simulink model "Q1"  (R2022b)
settings: Solver=VariableStepAuto  StartTime=0.0  StopTime=30  RelTol=1e-3
libraries: mpclib x5, slpidlib x3
settings Model: Creator=Alireza  LastModifiedBy=Alireza

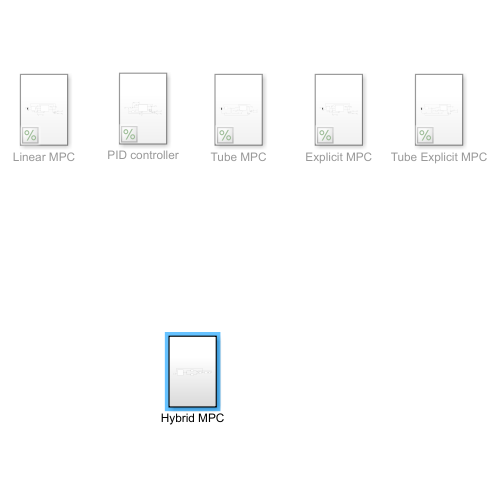
[thumbnail: Simulink's stored preview of the top-level diagram]
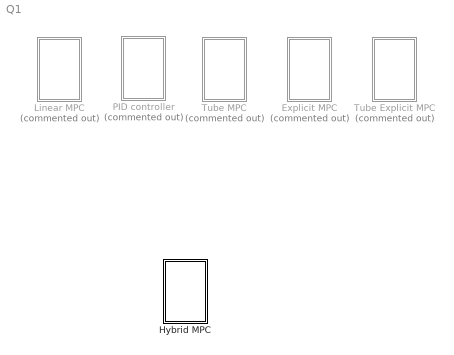
== system Q1 ==
  Explicit MPC : Subsystem  Commented=on
  Hybrid MPC : Subsystem
  Linear MPC : Subsystem  Commented=on
  PID controller : Subsystem  Commented=on
  Tube Explicit MPC : Subsystem  Commented=on
  Tube MPC : Subsystem  Commented=on

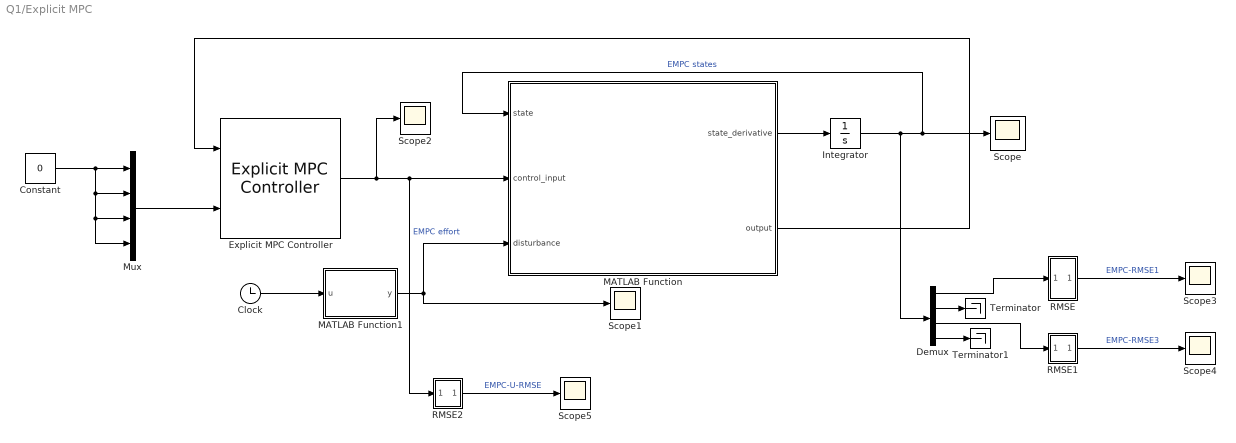
== system Q1/Explicit MPC ==
  Clock : Clock
  Constant : Constant  Value=0
  Demux : Demux
  Explicit MPC Controller : mpclib/Explicit MPC Controller  SCDEnableBlockLinearizationSpecification=on  empcobj=empc1  is_multiple=0  enable_value=0  return_u0=off  md_inport=off  mv_inport=off  return_status=off  return_region=off  return_state=off  state_inport=off  BlockDataType=double  SampleTimeInherited=off  switch_inport=off
  Integrator : Integrator  InitialCondition=[0;0;0;0]
  MATLAB Function : MATLAB Function  TreatAsAtomicUnit=on
  MATLAB Function1 : MATLAB Function  TreatAsAtomicUnit=on
  Mux : Mux
  RMSE : Subsystem
  RMSE1 : Subsystem
  RMSE2 : Subsystem
  Scope{,1..5} (6 alike) : Scope
  Terminator : Terminator
  Terminator1 : Terminator
  wires:
  RMSE/1(Out1) -> Scope3/1  "EMPC-RMSE1"
  MATLAB Function1/1(y) -> Scope1/1, MATLAB Function/3(disturbance)
  Constant/1 -> Mux/3, Mux/4, Mux/2, Mux/1
  Integrator/1 -> Demux/1, MATLAB Function/1(state), Scope/1  "EMPC states"
  Explicit MPC Controller/1 -> RMSE2/1(In1), MATLAB Function/2(control_input), Scope2/1  "EMPC effort"
  Demux/3 -> RMSE1/1(In1)
  Demux/2 -> Terminator/1
  Demux/4 -> Terminator1/1
  MATLAB Function/2(output) -> Explicit MPC Controller/1
  Demux/1 -> RMSE/1(In1)
  Mux/1 -> Explicit MPC Controller/2
  Clock/1 -> MATLAB Function1/1(u)
  MATLAB Function/1(state_derivative) -> Integrator/1
  RMSE1/1(Out1) -> Scope4/1  "EMPC-RMSE3"
  RMSE2/1(Out1) -> Scope5/1  "EMPC-U-RMSE"

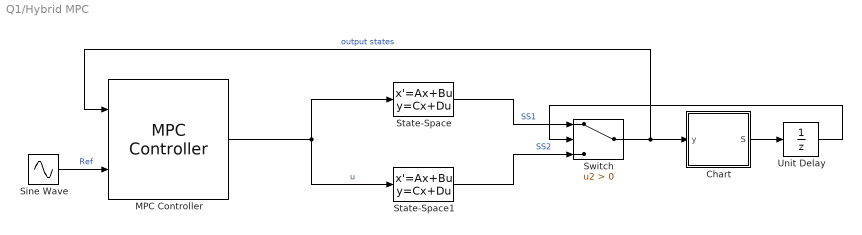
== system Q1/Hybrid MPC ==
  Chart : Stateflow chart  TreatAsAtomicUnit=on
  MPC Controller : mpclib/MPC Controller  SCDEnableBlockLinearizationSpecification=on  mpcobj=mpc1  is_multiple=0  enable_value=0  return_u0=off  updateMPCinCallerWorkspace=on  md_inport=off  mv_inport=off  uref_inport=off  return_cost=off  return_mvseq=off  return_qpstatus=off  return_xseq=off  return_state=off  return_ovseq=off  state_inport=off  umin_inport=off  umax_inport=off  ymin_inport=off  ymax_inport=off  cc_inport=off  ywt_inport=off  uwt_inport=off  duwt_inport=off  rhoeps_inport=off  pm_inport=off  MaximumP=10  HorizonChoice=FixedHorizon  n_ts=0.01  n_p=110  n_mv=1  n_md=0  n_ud=0  n_mo=1  n_uo=0  BlockDataType=double  SampleTimeInherited=off  switch_inport=off
  Sine Wave : Sin  Amplitude=20  Frequency=pi/10  SampleTime=0
  State-Space : StateSpace  A=[0 2;-2 -2]  B=[0;2]  C=[1 0]  D=[0]  InitialCondition=[0.5 ; 0]
  State-Space1 : StateSpace  A=[0 4;-4 -4]  B=[0;4]  C=[1 0]  D=[0]  InitialCondition=[0.5 ; 0]
  Switch : Switch  Criteria=u2 > Threshold  SaturateOnIntegerOverflow=off  InputSameDT=off
  Unit Delay : UnitDelay  SampleTime=-1  HasFrameUpgradeWarning=on
  wires:
  MPC Controller/1 -> State-Space1/1, State-Space/1  "u"
  State-Space1/1 -> Switch/3  "SS2"
  Switch/1 -> MPC Controller/1, Chart/1(y)  "output states"
  Sine Wave/1 -> MPC Controller/2  "Ref"
  State-Space/1 -> Switch/1  "SS1"
  Chart/1(S) -> Unit Delay/1
  Unit Delay/1 -> Switch/2

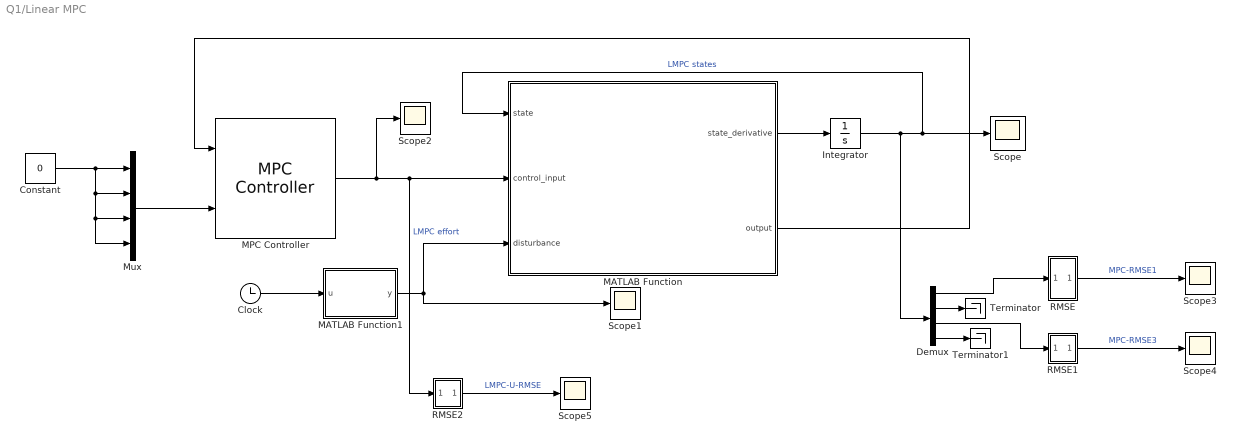
== system Q1/Linear MPC ==
  Clock : Clock
  Constant : Constant  Value=0
  Demux : Demux
  Integrator : Integrator  InitialCondition=[0;0;0;0]
  MATLAB Function : MATLAB Function  TreatAsAtomicUnit=on
  MATLAB Function1 : MATLAB Function  TreatAsAtomicUnit=on
  MPC Controller : mpclib/MPC Controller  SCDEnableBlockLinearizationSpecification=on  mpcobj=mpc1  is_multiple=0  enable_value=0  return_u0=off  updateMPCinCallerWorkspace=on  md_inport=off  mv_inport=off  uref_inport=off  return_cost=off  return_mvseq=off  return_qpstatus=off  return_xseq=off  return_state=off  return_ovseq=off  state_inport=off  umin_inport=off  umax_inport=off  ymin_inport=off  ymax_inport=off  cc_inport=off  ywt_inport=off  uwt_inport=off  duwt_inport=off  rhoeps_inport=off  pm_inport=off  MaximumP=10  HorizonChoice=FixedHorizon  n_ts=0.01  n_p=100  n_mv=1  n_md=0  n_ud=0  n_mo=4  n_uo=0  BlockDataType=double  SampleTimeInherited=off  switch_inport=off
  Mux : Mux
  RMSE : Subsystem
  RMSE1 : Subsystem
  RMSE2 : Subsystem
  Scope{,1..5} (6 alike) : Scope
  Terminator : Terminator
  Terminator1 : Terminator
  wires:
  RMSE/1(Out1) -> Scope3/1  "MPC-RMSE1"
  MATLAB Function1/1(y) -> Scope1/1, MATLAB Function/3(disturbance)
  Constant/1 -> Mux/3, Mux/4, Mux/2, Mux/1
  Integrator/1 -> Demux/1, MATLAB Function/1(state), Scope/1  "LMPC states"
  MPC Controller/1 -> RMSE2/1(In1), MATLAB Function/2(control_input), Scope2/1  "LMPC effort"
  Demux/3 -> RMSE1/1(In1)
  Demux/2 -> Terminator/1
  Demux/4 -> Terminator1/1
  MATLAB Function/2(output) -> MPC Controller/1
  Demux/1 -> RMSE/1(In1)
  Mux/1 -> MPC Controller/2
  Clock/1 -> MATLAB Function1/1(u)
  MATLAB Function/1(state_derivative) -> Integrator/1
  RMSE1/1(Out1) -> Scope4/1  "MPC-RMSE3"
  RMSE2/1(Out1) -> Scope5/1  "LMPC-U-RMSE"

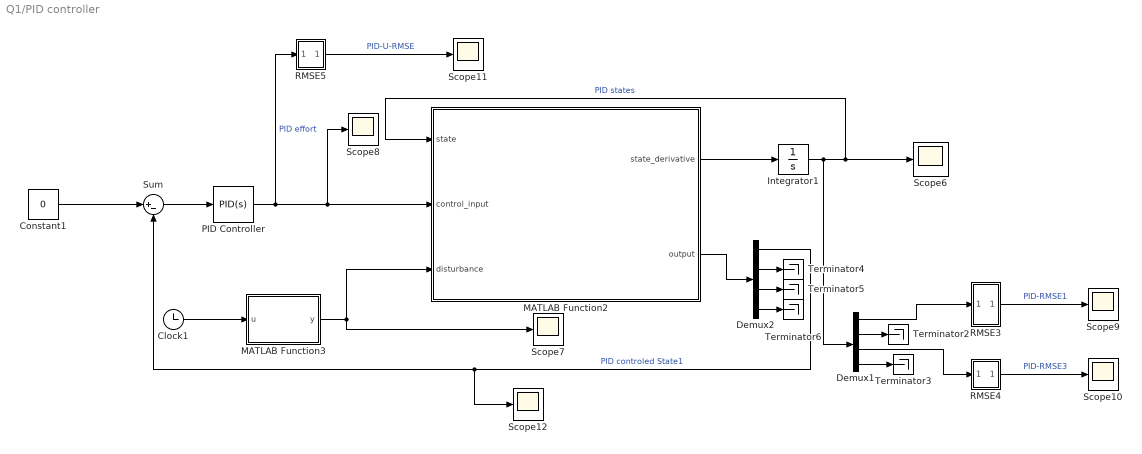
== system Q1/PID controller ==
  Clock1 : Clock
  Constant1 : Constant  Value=0
  Demux1 : Demux
  Demux2 : Demux
  Integrator1 : Integrator  InitialCondition=[0;0;0;0]
  MATLAB Function2 : MATLAB Function  TreatAsAtomicUnit=on
  MATLAB Function3 : MATLAB Function  TreatAsAtomicUnit=on
  PID Controller : slpidlib/PID Controller  Controller=PID  Form=Parallel  TimeDomain=Continuous-time  UseExternalTs=off  SampleTime=-1  IntegratorMethod=Forward Euler  FilterMethod=Forward Euler  ControllerParametersSource=internal  P=2115167.33224621  I=6808255.34812067  UseKiTs=off  D=134270.145058429  N=315.344677005256  UseFilter=on  TunerSelectOption=Transfer Function Based (PID Tuner App)  InitialConditionSource=internal  InitialConditionForIntegrator=0  InitialConditionForFilter=0  DifferentiatorICPrevScaledInput=0  ExternalReset=none  TrackingMode=off  Kt=1  LimitOutput=off  SatLimitsSource=internal  UpperSaturationLimit=inf  LowerSaturationLimit=-inf  LinearizeAsGain=on  AntiWindupMode=none  Kb=1  LimitIntegrator=off  UpperIntegratorSaturationLimit=inf  LowerIntegratorSaturationLimit=-inf  POutMin=[]  POutMax=[]  IOutMin=[]  IOutMax=[]  DOutMin=[]  DOutMax=[]  NOutMin=[]  NOutMax=[]  SumOutMin=[]  SumOutMax=[]  SaturationOutMin=[]  SaturationOutMax=[]  PParamMin=[]  PParamMax=[]  IParamMin=[]  IParamMax=[]  DParamMin=[]  DParamMax=[]  NParamMin=[]  NParamMax=[]  KbParamMin=[]  KbParamMax=[]  KtParamMin=[]  KtParamMax=[]  KbOutMin=[]  KbOutMax=[]  KtOutMin=[]  KtOutMax=[]  IntegratorOutMin=[]  IntegratorOutMax=[]  FilterOutMin=[]  FilterOutMax=[]  SumI1OutMin=[]  SumI1OutMax=[]  SumI2OutMin=[]  SumI2OutMax=[]  SumI3OutMin=[]  SumI3OutMax=[]  SumI4OutMin=[]  SumI4OutMax=[]  SumDOutMin=[]  SumDOutMax=[]  DifferentiatorOutMin=[]  DifferentiatorOutMax=[]  FilterDiffOutCoefMin=[]  FilterDiffOutCoefMax=[]  ReciprocalOutMin=[]  ReciprocalOutMax=[]  SumDenOutMin=[]  SumDenOutMax=[]  SumNumOutMin=[]  SumNumOutMax=[]  DivideOutMin=[]  DivideOutMax=[]  UdiffTsProdOutMin=[]  UdiffTsProdOutMax=[]  NTsProdOutMin=[]  NTsProdOutMax=[]  UintegralTsProdOutMin=[]  UintegralTsProdOutMax=[]  UngainTsProdOutMin=[]  UngainTsProdOutMax=[]  ClampingZeroOutDataTypeStr=Inherit: Inherit via back propagation  ClampingZeroOutMin=[]  ClampingZeroOutMax=[]  FilterDenConstantOutDataTypeStr=Inherit: Inherit via back propagation  FilterDenConstantOutMin=[]  FilterDenConstantOutMax=[]  PCopyOutDataTypeStr=Inherit: Inherit via back propagation  PCopyOutMin=[]  PCopyOutMax=[]  NCopyOutDataTypeStr=Inherit: Inherit via back propagation  NCopyOutMin=[]  NCopyOutMax=[]  IntegratorContinuousStateAttributes=''  IntegratorStateMustResolveToSignalObject=off  IntegratorRTWStateStorageClass=Auto  FilterContinuousStateAttributes=''  FilterStateMustResolveToSignalObject=off  FilterRTWStateStorageClass=Auto  ParallelPVariant=InternalParameters  IdealPVariant=Disabled  IVariant=InternalParameters  DVariant=InternalParameters  IntegratorVariant=Continuous  SatVariant=Disabled  AWVariant=Passthrough  PCopyVariant=Disabled  TRVariant=Disabled  FdbkBlocksVariant=Forward  IdealPFdbkVariant=Disabled  SatFdbkVariant=Disabled  DerivativeFilterVariant=ContFilter  NVariant=InternalParameters  NCopyVariant=Disabled  FilterICVariant=InternalICsFilter  IntegratorICVariant=InternalICs  ExternalResetVariant=Disabled  TRSumVariant=Passthrough  SumFdbkVariant=Disabled  SumVariant=Sum_PID  TsampFilterVariant=InternalTs  TsampNgainVariant=Passthrough  TsampIntegralVariant=Passthrough  ExternalSaturationOutDataTypeStr=Inherit: Same as second input
  RMSE3 : Subsystem
  RMSE4 : Subsystem
  RMSE5 : Subsystem
  Scope{6..12} (7 alike) : Scope
  Sum : Sum  Inputs=|+-
  Terminator{2..6} (5 alike) : Terminator
  wires:
  Demux2/4 -> Terminator6/1
  MATLAB Function3/1(y) -> Scope7/1, MATLAB Function2/3(disturbance)
  RMSE4/1(Out1) -> Scope10/1  "PID-RMSE3"
  Demux1/1 -> RMSE3/1(In1)
  Demux2/2 -> Terminator4/1
  Demux2/1 -> Scope12/1, Sum/2  "PID controled State1"
  PID Controller/1 -> Scope8/1, MATLAB Function2/2(control_input), RMSE5/1(In1)  "PID effort"
  MATLAB Function2/1(state_derivative) -> Integrator1/1
  Sum/1 -> PID Controller/1
  RMSE5/1(Out1) -> Scope11/1  "PID-U-RMSE"
  Integrator1/1 -> Demux1/1, MATLAB Function2/1(state), Scope6/1  "PID states"
  Constant1/1 -> Sum/1
  Demux1/2 -> Terminator2/1
  Demux1/4 -> Terminator3/1
  Clock1/1 -> MATLAB Function3/1(u)
  Demux1/3 -> RMSE4/1(In1)
  RMSE3/1(Out1) -> Scope9/1  "PID-RMSE1"
  MATLAB Function2/2(output) -> Demux2/1
  Demux2/3 -> Terminator5/1

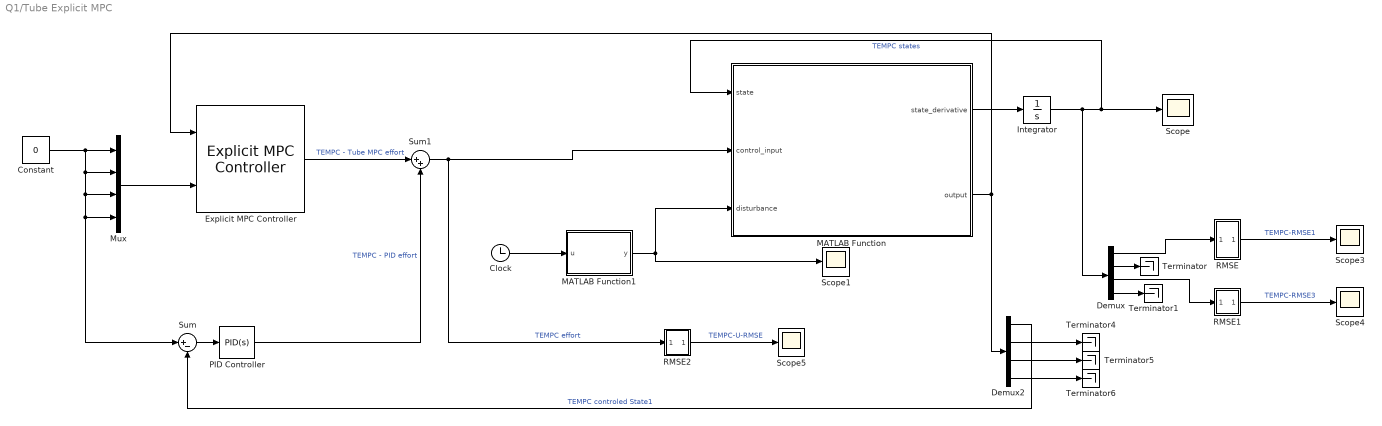
== system Q1/Tube Explicit MPC ==
  Clock : Clock
  Constant : Constant  Value=0
  Demux : Demux
  Demux2 : Demux
  Explicit MPC Controller : mpclib/Explicit MPC Controller  SCDEnableBlockLinearizationSpecification=on  empcobj=empc1  is_multiple=0  enable_value=0  return_u0=off  md_inport=off  mv_inport=off  return_status=off  return_region=off  return_state=off  state_inport=off  BlockDataType=double  SampleTimeInherited=off  switch_inport=off
  Integrator : Integrator  InitialCondition=[0;0;0;0]
  MATLAB Function : MATLAB Function  TreatAsAtomicUnit=on
  MATLAB Function1 : MATLAB Function  TreatAsAtomicUnit=on
  Mux : Mux
  PID Controller : slpidlib/PID Controller  Controller=PID  Form=Parallel  TimeDomain=Continuous-time  UseExternalTs=off  SampleTime=-1  IntegratorMethod=Forward Euler  FilterMethod=Forward Euler  ControllerParametersSource=internal  P=673792.542179079  I=2194376.82779204  UseKiTs=off  D=50799.688193398  N=2414.22496661449  UseFilter=on  TunerSelectOption=Transfer Function Based (PID Tuner App)  InitialConditionSource=internal  InitialConditionForIntegrator=0  InitialConditionForFilter=0  DifferentiatorICPrevScaledInput=0  ExternalReset=none  TrackingMode=off  Kt=1  LimitOutput=off  SatLimitsSource=internal  UpperSaturationLimit=inf  LowerSaturationLimit=-inf  LinearizeAsGain=on  AntiWindupMode=none  Kb=1  LimitIntegrator=off  UpperIntegratorSaturationLimit=inf  LowerIntegratorSaturationLimit=-inf  POutMin=[]  POutMax=[]  IOutMin=[]  IOutMax=[]  DOutMin=[]  DOutMax=[]  NOutMin=[]  NOutMax=[]  SumOutMin=[]  SumOutMax=[]  SaturationOutMin=[]  SaturationOutMax=[]  PParamMin=[]  PParamMax=[]  IParamMin=[]  IParamMax=[]  DParamMin=[]  DParamMax=[]  NParamMin=[]  NParamMax=[]  KbParamMin=[]  KbParamMax=[]  KtParamMin=[]  KtParamMax=[]  KbOutMin=[]  KbOutMax=[]  KtOutMin=[]  KtOutMax=[]  IntegratorOutMin=[]  IntegratorOutMax=[]  FilterOutMin=[]  FilterOutMax=[]  SumI1OutMin=[]  SumI1OutMax=[]  SumI2OutMin=[]  SumI2OutMax=[]  SumI3OutMin=[]  SumI3OutMax=[]  SumI4OutMin=[]  SumI4OutMax=[]  SumDOutMin=[]  SumDOutMax=[]  DifferentiatorOutMin=[]  DifferentiatorOutMax=[]  FilterDiffOutCoefMin=[]  FilterDiffOutCoefMax=[]  ReciprocalOutMin=[]  ReciprocalOutMax=[]  SumDenOutMin=[]  SumDenOutMax=[]  SumNumOutMin=[]  SumNumOutMax=[]  DivideOutMin=[]  DivideOutMax=[]  UdiffTsProdOutMin=[]  UdiffTsProdOutMax=[]  NTsProdOutMin=[]  NTsProdOutMax=[]  UintegralTsProdOutMin=[]  UintegralTsProdOutMax=[]  UngainTsProdOutMin=[]  UngainTsProdOutMax=[]  ClampingZeroOutDataTypeStr=Inherit: Inherit via back propagation  ClampingZeroOutMin=[]  ClampingZeroOutMax=[]  FilterDenConstantOutDataTypeStr=Inherit: Inherit via back propagation  FilterDenConstantOutMin=[]  FilterDenConstantOutMax=[]  PCopyOutDataTypeStr=Inherit: Inherit via back propagation  PCopyOutMin=[]  PCopyOutMax=[]  NCopyOutDataTypeStr=Inherit: Inherit via back propagation  NCopyOutMin=[]  NCopyOutMax=[]  IntegratorContinuousStateAttributes=''  IntegratorStateMustResolveToSignalObject=off  IntegratorRTWStateStorageClass=Auto  FilterContinuousStateAttributes=''  FilterStateMustResolveToSignalObject=off  FilterRTWStateStorageClass=Auto  ParallelPVariant=InternalParameters  IdealPVariant=Disabled  IVariant=InternalParameters  DVariant=InternalParameters  IntegratorVariant=Continuous  SatVariant=Disabled  AWVariant=Passthrough  PCopyVariant=Disabled  TRVariant=Disabled  FdbkBlocksVariant=Forward  IdealPFdbkVariant=Disabled  SatFdbkVariant=Disabled  DerivativeFilterVariant=ContFilter  NVariant=InternalParameters  NCopyVariant=Disabled  FilterICVariant=InternalICsFilter  IntegratorICVariant=InternalICs  ExternalResetVariant=Disabled  TRSumVariant=Passthrough  SumFdbkVariant=Disabled  SumVariant=Sum_PID  TsampFilterVariant=InternalTs  TsampNgainVariant=Passthrough  TsampIntegralVariant=Passthrough  ExternalSaturationOutDataTypeStr=Inherit: Same as second input
  RMSE : Subsystem
  RMSE1 : Subsystem
  RMSE2 : Subsystem
  Scope{,1,3..5} (5 alike) : Scope
  Sum : Sum  Inputs=|+-
  Sum1 : Sum  Inputs=|++
  Terminator{,1,4..6} (5 alike) : Terminator
  wires:
  PID Controller/1 -> Sum1/2  "TEMPC - PID effort"
  Demux2/1 -> Sum/2  "TEMPC controled State1"
  Sum/1 -> PID Controller/1
  MATLAB Function/2(output) -> Explicit MPC Controller/1, Demux2/1
  Demux2/4 -> Terminator6/1
  Demux2/3 -> Terminator5/1
  Demux2/2 -> Terminator4/1
  Sum1/1 -> MATLAB Function/2(control_input), RMSE2/1(In1)  "TEMPC effort"
  Explicit MPC Controller/1 -> Sum1/1  "TEMPC - Tube MPC effort"
  RMSE/1(Out1) -> Scope3/1  "TEMPC-RMSE1"
  MATLAB Function1/1(y) -> Scope1/1, MATLAB Function/3(disturbance)
  Constant/1 -> Mux/3, Mux/4, Sum/1, Mux/2, Mux/1
  Integrator/1 -> Demux/1, MATLAB Function/1(state), Scope/1  "TEMPC states"
  Demux/3 -> RMSE1/1(In1)
  Demux/2 -> Terminator/1
  Demux/4 -> Terminator1/1
  Demux/1 -> RMSE/1(In1)
  Mux/1 -> Explicit MPC Controller/2
  Clock/1 -> MATLAB Function1/1(u)
  MATLAB Function/1(state_derivative) -> Integrator/1
  RMSE1/1(Out1) -> Scope4/1  "TEMPC-RMSE3"
  RMSE2/1(Out1) -> Scope5/1  "TEMPC-U-RMSE"

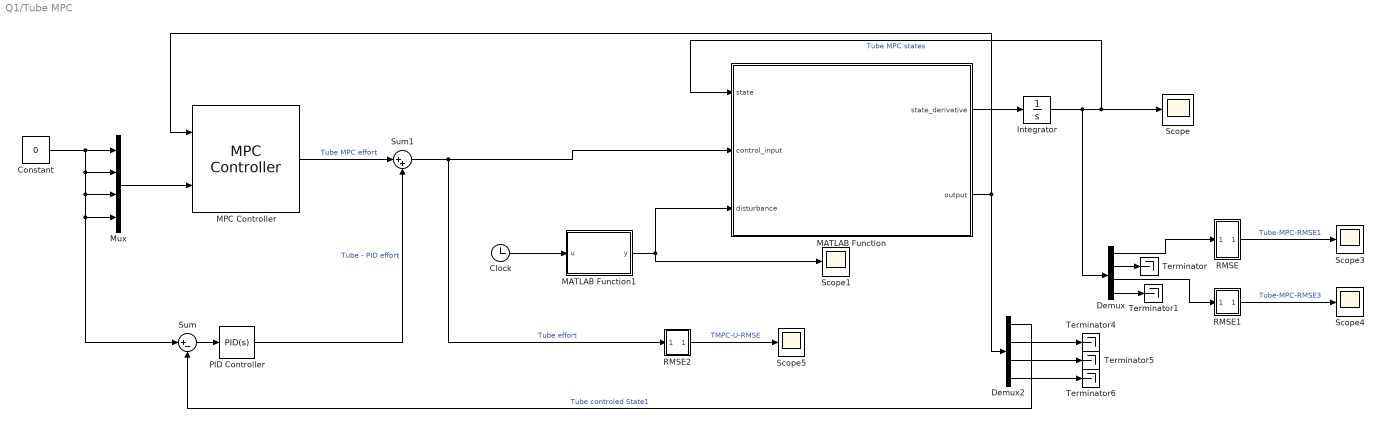
== system Q1/Tube MPC ==
  Clock : Clock
  Constant : Constant  Value=0
  Demux : Demux
  Demux2 : Demux
  Integrator : Integrator  InitialCondition=[0;0;0;0]
  MATLAB Function : MATLAB Function  TreatAsAtomicUnit=on
  MATLAB Function1 : MATLAB Function  TreatAsAtomicUnit=on
  MPC Controller : mpclib/MPC Controller  SCDEnableBlockLinearizationSpecification=on  mpcobj=mpc1  is_multiple=0  enable_value=0  return_u0=off  updateMPCinCallerWorkspace=on  md_inport=off  mv_inport=off  uref_inport=off  return_cost=off  return_mvseq=off  return_qpstatus=off  return_xseq=off  return_state=off  return_ovseq=off  state_inport=off  umin_inport=off  umax_inport=off  ymin_inport=off  ymax_inport=off  cc_inport=off  ywt_inport=off  uwt_inport=off  duwt_inport=off  rhoeps_inport=off  pm_inport=off  MaximumP=10  HorizonChoice=FixedHorizon  n_ts=0.01  n_p=100  n_mv=1  n_md=0  n_ud=0  n_mo=4  n_uo=0  BlockDataType=double  SampleTimeInherited=off  switch_inport=off
  Mux : Mux
  PID Controller : slpidlib/PID Controller  Controller=PID  Form=Parallel  TimeDomain=Continuous-time  UseExternalTs=off  SampleTime=-1  IntegratorMethod=Forward Euler  FilterMethod=Forward Euler  ControllerParametersSource=internal  P=673792.542179079  I=2194376.82779204  UseKiTs=off  D=50799.688193398  N=2414.22496661449  UseFilter=on  TunerSelectOption=Transfer Function Based (PID Tuner App)  InitialConditionSource=internal  InitialConditionForIntegrator=0  InitialConditionForFilter=0  DifferentiatorICPrevScaledInput=0  ExternalReset=none  TrackingMode=off  Kt=1  LimitOutput=off  SatLimitsSource=internal  UpperSaturationLimit=inf  LowerSaturationLimit=-inf  LinearizeAsGain=on  AntiWindupMode=none  Kb=1  LimitIntegrator=off  UpperIntegratorSaturationLimit=inf  LowerIntegratorSaturationLimit=-inf  POutMin=[]  POutMax=[]  IOutMin=[]  IOutMax=[]  DOutMin=[]  DOutMax=[]  NOutMin=[]  NOutMax=[]  SumOutMin=[]  SumOutMax=[]  SaturationOutMin=[]  SaturationOutMax=[]  PParamMin=[]  PParamMax=[]  IParamMin=[]  IParamMax=[]  DParamMin=[]  DParamMax=[]  NParamMin=[]  NParamMax=[]  KbParamMin=[]  KbParamMax=[]  KtParamMin=[]  KtParamMax=[]  KbOutMin=[]  KbOutMax=[]  KtOutMin=[]  KtOutMax=[]  IntegratorOutMin=[]  IntegratorOutMax=[]  FilterOutMin=[]  FilterOutMax=[]  SumI1OutMin=[]  SumI1OutMax=[]  SumI2OutMin=[]  SumI2OutMax=[]  SumI3OutMin=[]  SumI3OutMax=[]  SumI4OutMin=[]  SumI4OutMax=[]  SumDOutMin=[]  SumDOutMax=[]  DifferentiatorOutMin=[]  DifferentiatorOutMax=[]  FilterDiffOutCoefMin=[]  FilterDiffOutCoefMax=[]  ReciprocalOutMin=[]  ReciprocalOutMax=[]  SumDenOutMin=[]  SumDenOutMax=[]  SumNumOutMin=[]  SumNumOutMax=[]  DivideOutMin=[]  DivideOutMax=[]  UdiffTsProdOutMin=[]  UdiffTsProdOutMax=[]  NTsProdOutMin=[]  NTsProdOutMax=[]  UintegralTsProdOutMin=[]  UintegralTsProdOutMax=[]  UngainTsProdOutMin=[]  UngainTsProdOutMax=[]  ClampingZeroOutDataTypeStr=Inherit: Inherit via back propagation  ClampingZeroOutMin=[]  ClampingZeroOutMax=[]  FilterDenConstantOutDataTypeStr=Inherit: Inherit via back propagation  FilterDenConstantOutMin=[]  FilterDenConstantOutMax=[]  PCopyOutDataTypeStr=Inherit: Inherit via back propagation  PCopyOutMin=[]  PCopyOutMax=[]  NCopyOutDataTypeStr=Inherit: Inherit via back propagation  NCopyOutMin=[]  NCopyOutMax=[]  IntegratorContinuousStateAttributes=''  IntegratorStateMustResolveToSignalObject=off  IntegratorRTWStateStorageClass=Auto  FilterContinuousStateAttributes=''  FilterStateMustResolveToSignalObject=off  FilterRTWStateStorageClass=Auto  ParallelPVariant=InternalParameters  IdealPVariant=Disabled  IVariant=InternalParameters  DVariant=InternalParameters  IntegratorVariant=Continuous  SatVariant=Disabled  AWVariant=Passthrough  PCopyVariant=Disabled  TRVariant=Disabled  FdbkBlocksVariant=Forward  IdealPFdbkVariant=Disabled  SatFdbkVariant=Disabled  DerivativeFilterVariant=ContFilter  NVariant=InternalParameters  NCopyVariant=Disabled  FilterICVariant=InternalICsFilter  IntegratorICVariant=InternalICs  ExternalResetVariant=Disabled  TRSumVariant=Passthrough  SumFdbkVariant=Disabled  SumVariant=Sum_PID  TsampFilterVariant=InternalTs  TsampNgainVariant=Passthrough  TsampIntegralVariant=Passthrough  ExternalSaturationOutDataTypeStr=Inherit: Same as second input
  RMSE : Subsystem
  RMSE1 : Subsystem
  RMSE2 : Subsystem
  Scope{,1,3..5} (5 alike) : Scope
  Sum : Sum  Inputs=|+-
  Sum1 : Sum  Inputs=|++
  Terminator{,1,4..6} (5 alike) : Terminator
  wires:
  RMSE2/1(Out1) -> Scope5/1  "TMPC-U-RMSE"
  RMSE1/1(Out1) -> Scope4/1  "Tube-MPC-RMSE3"
  MATLAB Function/1(state_derivative) -> Integrator/1
  Clock/1 -> MATLAB Function1/1(u)
  Mux/1 -> MPC Controller/2
  Demux/1 -> RMSE/1(In1)
  Demux/4 -> Terminator1/1
  Demux/2 -> Terminator/1
  Demux/3 -> RMSE1/1(In1)
  Integrator/1 -> Scope/1, MATLAB Function/1(state), Demux/1  "Tube MPC states"
  Constant/1 -> Mux/1, Mux/2, Sum/1, Mux/4, Mux/3
  MATLAB Function1/1(y) -> MATLAB Function/3(disturbance), Scope1/1
  RMSE/1(Out1) -> Scope3/1  "Tube-MPC-RMSE1"
  MPC Controller/1 -> Sum1/1  "Tube MPC effort"
  Sum1/1 -> RMSE2/1(In1), MATLAB Function/2(control_input)  "Tube effort"
  Demux2/2 -> Terminator4/1
  Demux2/3 -> Terminator5/1
  Demux2/4 -> Terminator6/1
  MATLAB Function/2(output) -> MPC Controller/1, Demux2/1
  Sum/1 -> PID Controller/1
  Demux2/1 -> Sum/2  "Tube controled State1"
  PID Controller/1 -> Sum1/2  "Tube - PID effort"

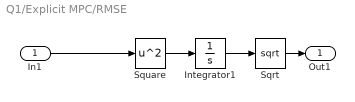
== system Q1/Explicit MPC/RMSE ==
  In1 : Inport
  Integrator1 : Integrator
  Sqrt : Sqrt
  Square : Math  Operator=square
  Out1 : Outport
  wires:
  Integrator1/1 -> Sqrt/1
  Square/1 -> Integrator1/1
  In1/1 -> Square/1
  Sqrt/1 -> Out1/1

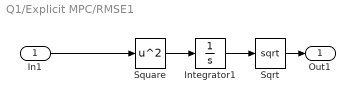
== system Q1/Explicit MPC/RMSE1 ==
  In1 : Inport
  Integrator1 : Integrator
  Sqrt : Sqrt
  Square : Math  Operator=square
  Out1 : Outport
  wires:
  Sqrt/1 -> Out1/1
  In1/1 -> Square/1
  Square/1 -> Integrator1/1
  Integrator1/1 -> Sqrt/1

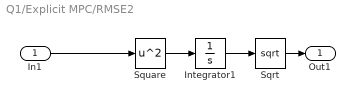
== system Q1/Explicit MPC/RMSE2 ==
  In1 : Inport
  Integrator1 : Integrator
  Sqrt : Sqrt
  Square : Math  Operator=square
  Out1 : Outport
  wires:
  Integrator1/1 -> Sqrt/1
  Square/1 -> Integrator1/1
  In1/1 -> Square/1
  Sqrt/1 -> Out1/1

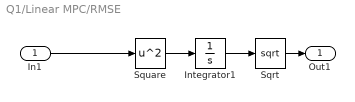
== system Q1/Linear MPC/RMSE ==
  In1 : Inport
  Integrator1 : Integrator
  Sqrt : Sqrt
  Square : Math  Operator=square
  Out1 : Outport
  wires:
  Integrator1/1 -> Sqrt/1
  Square/1 -> Integrator1/1
  In1/1 -> Square/1
  Sqrt/1 -> Out1/1

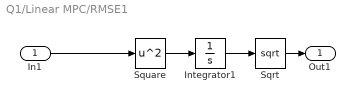
== system Q1/Linear MPC/RMSE1 ==
  In1 : Inport
  Integrator1 : Integrator
  Sqrt : Sqrt
  Square : Math  Operator=square
  Out1 : Outport
  wires:
  Sqrt/1 -> Out1/1
  In1/1 -> Square/1
  Square/1 -> Integrator1/1
  Integrator1/1 -> Sqrt/1

== system Q1/Linear MPC/RMSE2 ==
  In1 : Inport
  Integrator1 : Integrator
  Sqrt : Sqrt
  Square : Math  Operator=square
  Out1 : Outport
  wires:
  Integrator1/1 -> Sqrt/1
  Square/1 -> Integrator1/1
  In1/1 -> Square/1
  Sqrt/1 -> Out1/1

== system Q1/PID controller/RMSE3 ==
  In1 : Inport
  Integrator1 : Integrator
  Sqrt : Sqrt
  Square : Math  Operator=square
  Out1 : Outport
  wires:
  Integrator1/1 -> Sqrt/1
  Square/1 -> Integrator1/1
  In1/1 -> Square/1
  Sqrt/1 -> Out1/1

== system Q1/PID controller/RMSE4 ==
  In1 : Inport
  Integrator1 : Integrator
  Sqrt : Sqrt
  Square : Math  Operator=square
  Out1 : Outport
  wires:
  Sqrt/1 -> Out1/1
  In1/1 -> Square/1
  Square/1 -> Integrator1/1
  Integrator1/1 -> Sqrt/1

== system Q1/PID controller/RMSE5 ==
  In1 : Inport
  Integrator1 : Integrator
  Sqrt : Sqrt
  Square : Math  Operator=square
  Out1 : Outport
  wires:
  Integrator1/1 -> Sqrt/1
  Square/1 -> Integrator1/1
  In1/1 -> Square/1
  Sqrt/1 -> Out1/1

== system Q1/Tube Explicit MPC/RMSE ==
  In1 : Inport
  Integrator1 : Integrator
  Sqrt : Sqrt
  Square : Math  Operator=square
  Out1 : Outport
  wires:
  Integrator1/1 -> Sqrt/1
  Square/1 -> Integrator1/1
  In1/1 -> Square/1
  Sqrt/1 -> Out1/1

== system Q1/Tube Explicit MPC/RMSE1 ==
  In1 : Inport
  Integrator1 : Integrator
  Sqrt : Sqrt
  Square : Math  Operator=square
  Out1 : Outport
  wires:
  Sqrt/1 -> Out1/1
  In1/1 -> Square/1
  Square/1 -> Integrator1/1
  Integrator1/1 -> Sqrt/1

== system Q1/Tube Explicit MPC/RMSE2 ==
  In1 : Inport
  Integrator1 : Integrator
  Sqrt : Sqrt
  Square : Math  Operator=square
  Out1 : Outport
  wires:
  Integrator1/1 -> Sqrt/1
  Square/1 -> Integrator1/1
  In1/1 -> Square/1
  Sqrt/1 -> Out1/1

== system Q1/Tube MPC/RMSE ==
  In1 : Inport
  Integrator1 : Integrator
  Sqrt : Sqrt
  Square : Math  Operator=square
  Out1 : Outport
  wires:
  Sqrt/1 -> Out1/1
  In1/1 -> Square/1
  Square/1 -> Integrator1/1
  Integrator1/1 -> Sqrt/1

== system Q1/Tube MPC/RMSE1 ==
  In1 : Inport
  Integrator1 : Integrator
  Sqrt : Sqrt
  Square : Math  Operator=square
  Out1 : Outport
  wires:
  Integrator1/1 -> Sqrt/1
  Square/1 -> Integrator1/1
  In1/1 -> Square/1
  Sqrt/1 -> Out1/1

== system Q1/Tube MPC/RMSE2 ==
  In1 : Inport
  Integrator1 : Integrator
  Sqrt : Sqrt
  Square : Math  Operator=square
  Out1 : Outport
  wires:
  Sqrt/1 -> Out1/1
  In1/1 -> Square/1
  Square/1 -> Integrator1/1
  Integrator1/1 -> Sqrt/1

== matlab function Q1/Linear MPC/MATLAB Function1 ==
  data: u input; y output
function y = distrubance(u)

if u>=4 & u<5
    y = (u-4);
elseif u>=5 & u<= 7
    y = 1;
elseif u>7 & u<8
    y = -u+8;
else
    y = 0;
end

== matlab function Q1/Linear MPC/MATLAB Function ==
  data: state input; control_input input; state_derivative output; disturbance input; output output
function [state_derivative, output] = vehicle_suspension_dynamics(state, control_input, disturbance)
    % Parameters of the suspension system
    sprung_mass = 2500;    % Sprung mass (kg)
    unsprung_mass = 320;   % Unsprung mass (kg)
    spring_constant_s = 80000;  % Spring constant of the suspension (N/m)
    spring_constant_u = 500000; % Spring constant of the tire (N/m)
    damping_coefficient_s = 350;   % Damping coefficient of the suspension (Ns/m)
    damping_coefficient_u = 15020; % Damping coefficient of the tire (Ns/m)

    % State-space matrices
    % State vector: [x_s; v_s; x_u; v_u]
    % x_s: Displacement of the sprung mass
    % v_s: Velocity of the sprung mass
    % x_u: Displacement of the unsprung mass
    % v_u: Velocity of the unsprung mass

    A_matrix = [
        0,                      1,                      0,                      0;
        0,  -damping_coefficient_s/sprung_mass, -spring_constant_s/sprung_mass,  damping_coefficient_s/sprung_mass;
        0,                      1,                      0,                     -1;
       -spring_constant_u/unsprung_mass, damping_coefficient_s/unsprung_mass, (spring_constant_s + spring_constant_u)/unsprung_mass, -(damping_coefficient_s + damping_coefficient_u)/unsprung_mass
    ];

    % Input matrices
    B_disturbance = [
        0;
        damping_coefficient_s * damping_coefficient_u / (sprung_mass * unsprung_mass);
       -damping_coefficient_u / unsprung_mass;
        damping_coefficient_u / unsprung_mass * (spring_constant_u / damping_coefficient_u - damping_coefficient_s / unsprung_mass - damping_coefficient_u / unsprung_mass)
    ];

    B_control = [
        0;
        1 / sprung_mass;
        0;
       -1 / unsprung_mass
    ];

    % Compute state derivative
    state_derivative = A_matrix * state + B_disturbance * disturbance + B_control * control_input;

    % Compute output vector
    % Output vector is [x_s; v_s; x_u; placeholder], where placeholder is fixed at 0
    output = zeros(4, 1);
    output(1) = state(1);  % Sprung mass displacement
    output(2) = state(2);  % Sprung mass velocity
    output(3) = state(3);  % Unsprung mass displacement
    output(4) = 0;         % Placeholder
end

== matlab function Q1/PID controller/MATLAB Function2 ==
  data: state input; control_input input; state_derivative output; disturbance input; output output
function [state_derivative, output] = vehicle_suspension_dynamics(state, control_input, disturbance)
    % Parameters of the suspension system
    sprung_mass = 2500;    % Sprung mass (kg)
    unsprung_mass = 320;   % Unsprung mass (kg)
    spring_constant_s = 80000;  % Spring constant of the suspension (N/m)
    spring_constant_u = 500000; % Spring constant of the tire (N/m)
    damping_coefficient_s = 350;   % Damping coefficient of the suspension (Ns/m)
    damping_coefficient_u = 15020; % Damping coefficient of the tire (Ns/m)

    % State-space matrices
    % State vector: [x_s; v_s; x_u; v_u]
    % x_s: Displacement of the sprung mass
    % v_s: Velocity of the sprung mass
    % x_u: Displacement of the unsprung mass
    % v_u: Velocity of the unsprung mass

    A_matrix = [
        0,                      1,                      0,                      0;
        0,  -damping_coefficient_s/sprung_mass, -spring_constant_s/sprung_mass,  damping_coefficient_s/sprung_mass;
        0,                      1,                      0,                     -1;
       -spring_constant_u/unsprung_mass, damping_coefficient_s/unsprung_mass, (spring_constant_s + spring_constant_u)/unsprung_mass, -(damping_coefficient_s + damping_coefficient_u)/unsprung_mass
    ];

    % Input matrices
    B_disturbance = [
        0;
        damping_coefficient_s * damping_coefficient_u / (sprung_mass * unsprung_mass);
       -damping_coefficient_u / unsprung_mass;
        damping_coefficient_u / unsprung_mass * (spring_constant_u / damping_coefficient_u - damping_coefficient_s / unsprung_mass - damping_coefficient_u / unsprung_mass)
    ];

    B_control = [
        0;
        1 / sprung_mass;
        0;
       -1 / unsprung_mass
    ];

    % Compute state derivative
    state_derivative = A_matrix * state + B_disturbance * disturbance + B_control * control_input;

    % Compute output vector
    % Output vector is [x_s; v_s; x_u; placeholder], where placeholder is fixed at 0
    output = zeros(4, 1);
    output(1) = state(1);  % Sprung mass displacement
    output(2) = state(2);  % Sprung mass velocity
    output(3) = state(3);  % Unsprung mass displacement
    output(4) = 0;         % Placeholder
end

== matlab function Q1/PID controller/MATLAB Function3 ==
  data: u input; y output
function y = distrubance(u)

if u>=4 & u<5
    y = (u-4);
elseif u>=5 & u<= 7
    y = 1;
elseif u>7 & u<8
    y = -u+8;
else
    y = 0;
end

== matlab function Q1/Explicit MPC/MATLAB Function ==
  data: state input; control_input input; state_derivative output; disturbance input; output output
function [state_derivative, output] = vehicle_suspension_dynamics(state, control_input, disturbance)
    % Parameters of the suspension system
    sprung_mass = 2500;    % Sprung mass (kg)
    unsprung_mass = 320;   % Unsprung mass (kg)
    spring_constant_s = 80000;  % Spring constant of the suspension (N/m)
    spring_constant_u = 500000; % Spring constant of the tire (N/m)
    damping_coefficient_s = 350;   % Damping coefficient of the suspension (Ns/m)
    damping_coefficient_u = 15020; % Damping coefficient of the tire (Ns/m)

    % State-space matrices
    % State vector: [x_s; v_s; x_u; v_u]
    % x_s: Displacement of the sprung mass
    % v_s: Velocity of the sprung mass
    % x_u: Displacement of the unsprung mass
    % v_u: Velocity of the unsprung mass

    A_matrix = [
        0,                      1,                      0,                      0;
        0,  -damping_coefficient_s/sprung_mass, -spring_constant_s/sprung_mass,  damping_coefficient_s/sprung_mass;
        0,                      1,                      0,                     -1;
       -spring_constant_u/unsprung_mass, damping_coefficient_s/unsprung_mass, (spring_constant_s + spring_constant_u)/unsprung_mass, -(damping_coefficient_s + damping_coefficient_u)/unsprung_mass
    ];

    % Input matrices
    B_disturbance = [
        0;
        damping_coefficient_s * damping_coefficient_u / (sprung_mass * unsprung_mass);
       -damping_coefficient_u / unsprung_mass;
        damping_coefficient_u / unsprung_mass * (spring_constant_u / damping_coefficient_u - damping_coefficient_s / unsprung_mass - damping_coefficient_u / unsprung_mass)
    ];

    B_control = [
        0;
        1 / sprung_mass;
        0;
       -1 / unsprung_mass
    ];

    % Compute state derivative
    state_derivative = A_matrix * state + B_disturbance * disturbance + B_control * control_input;

    % Compute output vector
    % Output vector is [x_s; v_s; x_u; placeholder], where placeholder is fixed at 0
    output = zeros(4, 1);
    output(1) = state(1);  % Sprung mass displacement
    output(2) = state(2);  % Sprung mass velocity
    output(3) = state(3);  % Unsprung mass displacement
    output(4) = 0;         % Placeholder
end

== matlab function Q1/Explicit MPC/MATLAB Function1 ==
  data: u input; y output
function y = distrubance(u)

if u>=4 & u<5
    y = (u-4);
elseif u>=5 & u<= 7
    y = 1;
elseif u>7 & u<8
    y = -u+8;
else
    y = 0;
end

== matlab function Q1/Tube MPC/MATLAB Function ==
  data: state input; control_input input; state_derivative output; disturbance input; output output
function [state_derivative, output] = vehicle_suspension_dynamics(state, control_input, disturbance)
    % Parameters of the suspension system
    sprung_mass = 2500;    % Sprung mass (kg)
    unsprung_mass = 320;   % Unsprung mass (kg)
    spring_constant_s = 80000;  % Spring constant of the suspension (N/m)
    spring_constant_u = 500000; % Spring constant of the tire (N/m)
    damping_coefficient_s = 350;   % Damping coefficient of the suspension (Ns/m)
    damping_coefficient_u = 15020; % Damping coefficient of the tire (Ns/m)

    % State-space matrices
    % State vector: [x_s; v_s; x_u; v_u]
    % x_s: Displacement of the sprung mass
    % v_s: Velocity of the sprung mass
    % x_u: Displacement of the unsprung mass
    % v_u: Velocity of the unsprung mass

    A_matrix = [
        0,                      1,                      0,                      0;
        0,  -damping_coefficient_s/sprung_mass, -spring_constant_s/sprung_mass,  damping_coefficient_s/sprung_mass;
        0,                      1,                      0,                     -1;
       -spring_constant_u/unsprung_mass, damping_coefficient_s/unsprung_mass, (spring_constant_s + spring_constant_u)/unsprung_mass, -(damping_coefficient_s + damping_coefficient_u)/unsprung_mass
    ];

    % Input matrices
    B_disturbance = [
        0;
        damping_coefficient_s * damping_coefficient_u / (sprung_mass * unsprung_mass);
       -damping_coefficient_u / unsprung_mass;
        damping_coefficient_u / unsprung_mass * (spring_constant_u / damping_coefficient_u - damping_coefficient_s / unsprung_mass - damping_coefficient_u / unsprung_mass)
    ];

    B_control = [
        0;
        1 / sprung_mass;
        0;
       -1 / unsprung_mass
    ];

    % Compute state derivative
    state_derivative = A_matrix * state + B_disturbance * disturbance + B_control * control_input;

    % Compute output vector
    % Output vector is [x_s; v_s; x_u; placeholder], where placeholder is fixed at 0
    output = zeros(4, 1);
    output(1) = state(1);  % Sprung mass displacement
    output(2) = state(2);  % Sprung mass velocity
    output(3) = state(3);  % Unsprung mass displacement
    output(4) = 0;         % Placeholder
end

== matlab function Q1/Tube MPC/MATLAB Function1 ==
  data: u input; y output
function y = distrubance(u)

if u>=4 & u<5
    y = (u-4);
elseif u>=5 & u<= 7
    y = 1;
elseif u>7 & u<8
    y = -u+8;
else
    y = 0;
end

== matlab function Q1/Tube Explicit MPC/MATLAB Function ==
  data: state input; control_input input; state_derivative output; disturbance input; output output
function [state_derivative, output] = vehicle_suspension_dynamics(state, control_input, disturbance)
    % Parameters of the suspension system
    sprung_mass = 2500;    % Sprung mass (kg)
    unsprung_mass = 320;   % Unsprung mass (kg)
    spring_constant_s = 80000;  % Spring constant of the suspension (N/m)
    spring_constant_u = 500000; % Spring constant of the tire (N/m)
    damping_coefficient_s = 350;   % Damping coefficient of the suspension (Ns/m)
    damping_coefficient_u = 15020; % Damping coefficient of the tire (Ns/m)

    % State-space matrices
    % State vector: [x_s; v_s; x_u; v_u]
    % x_s: Displacement of the sprung mass
    % v_s: Velocity of the sprung mass
    % x_u: Displacement of the unsprung mass
    % v_u: Velocity of the unsprung mass

    A_matrix = [
        0,                      1,                      0,                      0;
        0,  -damping_coefficient_s/sprung_mass, -spring_constant_s/sprung_mass,  damping_coefficient_s/sprung_mass;
        0,                      1,                      0,                     -1;
       -spring_constant_u/unsprung_mass, damping_coefficient_s/unsprung_mass, (spring_constant_s + spring_constant_u)/unsprung_mass, -(damping_coefficient_s + damping_coefficient_u)/unsprung_mass
    ];

    % Input matrices
    B_disturbance = [
        0;
        damping_coefficient_s * damping_coefficient_u / (sprung_mass * unsprung_mass);
       -damping_coefficient_u / unsprung_mass;
        damping_coefficient_u / unsprung_mass * (spring_constant_u / damping_coefficient_u - damping_coefficient_s / unsprung_mass - damping_coefficient_u / unsprung_mass)
    ];

    B_control = [
        0;
        1 / sprung_mass;
        0;
       -1 / unsprung_mass
    ];

    % Compute state derivative
    state_derivative = A_matrix * state + B_disturbance * disturbance + B_control * control_input;

    % Compute output vector
    % Output vector is [x_s; v_s; x_u; placeholder], where placeholder is fixed at 0
    output = zeros(4, 1);
    output(1) = state(1);  % Sprung mass displacement
    output(2) = state(2);  % Sprung mass velocity
    output(3) = state(3);  % Unsprung mass displacement
    output(4) = 0;         % Placeholder
end

== matlab function Q1/Tube Explicit MPC/MATLAB Function1 ==
  data: u input; y output
function y = distrubance(u)

if u>=4 & u<5
    y = (u-4);
elseif u>=5 & u<= 7
    y = 1;
elseif u>7 & u<8
    y = -u+8;
else
    y = 0;
end

== stateflow chart Q1/Hybrid MPC/Chart ==
  state Mode1
    en: S=1
  state Mode2
    en:S=0
  (default) -> Mode1
  Mode1 -> Mode2 : [y>5]
  Mode2 -> Mode1 : [y<-5]
  data: y input; S output
